simulink model "modelsimulink"  (R2025b)
settings: Solver=VariableStepAuto  StartTime=0.0  StopTime=10  RelTol=1e-3
settings Model: Creator=nuris  LastModifiedBy=nuris

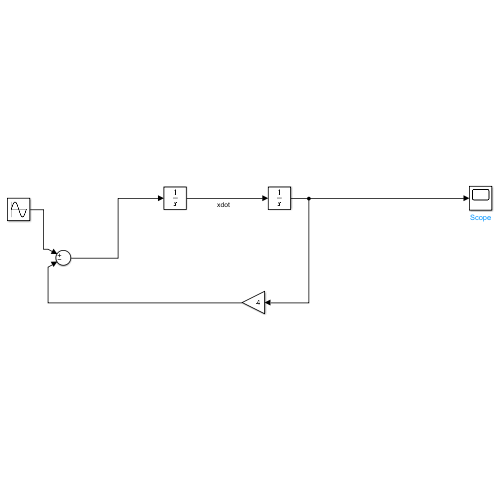
[thumbnail: Simulink's stored preview of the top-level diagram]
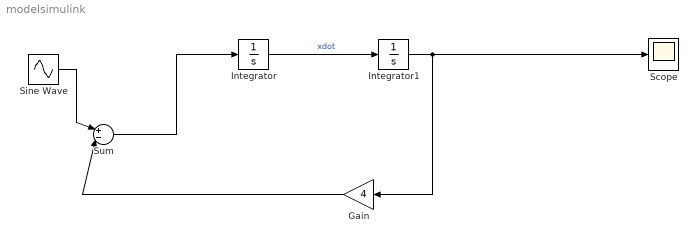
== system modelsimulink ==
  Gain : Gain  Gain=4
  Integrator : Integrator  InitialCondition=-3
  Integrator1 : Integrator  InitialCondition=5
  Scope : Scope
      settings: ActiveDisplayYMinimum=-3.9499936036533674  ActiveDisplayYMaximum=5.9944437337392626
  Sine Wave : Sin  Amplitude=2  Frequency=3  SampleTime=0
  Sum : Sum  Inputs=|+-|
  wires:
  Integrator/1 -> Integrator1/1  "xdot"
  Integrator1/1 -> Gain/1, Scope/1
  Sine Wave/1 -> Sum/1
  Gain/1 -> Sum/2
  Sum/1 -> Integrator/1
